simulink model "ppsim"  (R2024b)
settings: Solver=VariableStepAuto  StartTime=0.0  StopTime=10.0  RelTol=1e-3
values from neighbouring files (symbols this model uses):
  PpARMAXReg = ppc(tfarmax, ones(1, 4) * 0.3)    [main.m]
  PpARXReg = ppc(tfarx, ones(1, 4) * 0.3)    [main.m]
  PpDTFReg = ppc(dtf, ones(1, 4) * 0.1)    [main.m]
  usim = 1    [main.m]
  ut = [1 5]    [main.m]
undefined symbols (not defined in the file or in its folder): dtf, tfarmax, tfarx
settings Model: Creator=markminerov  LastModifiedBy=markminerov
settings DebuggingCC: AlgebraicLoopMsg=none

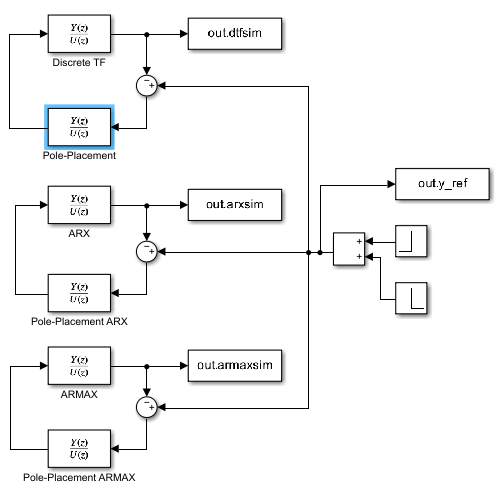
[thumbnail: Simulink's stored preview of the top-level diagram]
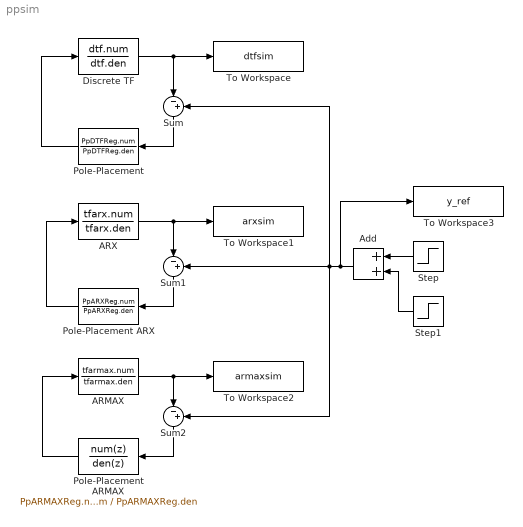
== system ppsim ==
  ARMAX : DiscreteTransferFcn  Numerator=tfarmax.num  Denominator=tfarmax.den
  ARX : DiscreteTransferFcn  Numerator=tfarx.num  Denominator=tfarx.den
  Add : Sum
  Discrete TF : DiscreteTransferFcn  Numerator=dtf.num  Denominator=dtf.den
  Pole-Placement : DiscreteTransferFcn  Numerator=PpDTFReg.num  Denominator=PpDTFReg.den
  Pole-Placement ARMAX : DiscreteTransferFcn  Numerator=PpARMAXReg.num  Denominator=PpARMAXReg.den
  Pole-Placement ARX : DiscreteTransferFcn  Numerator=PpARXReg.num  Denominator=PpARXReg.den
  Step : Step  Time=ut(1)  After=usim  SampleTime=0
  Step1 : Step  Time=ut(2)  After=-usim  SampleTime=0
  Sum : Sum  Inputs=|-+
  Sum1 : Sum  Inputs=|-+
  Sum2 : Sum  Inputs=|-+
  To Workspace : ToWorkspace  VariableName=dtfsim  SaveFormat=Timeseries  SampleTime=-1
  To Workspace1 : ToWorkspace  VariableName=arxsim  SaveFormat=Timeseries  SampleTime=-1
  To Workspace2 : ToWorkspace  VariableName=armaxsim  SaveFormat=Timeseries  SampleTime=-1
  To Workspace3 : ToWorkspace  VariableName=y_ref  SaveFormat=Timeseries  SampleTime=-1
  wires:
  Pole-Placement ARMAX/1 -> ARMAX/1
  Sum2/1 -> Pole-Placement ARMAX/1
  ARMAX/1 -> To Workspace2/1, Sum2/1
  Sum/1 -> Pole-Placement/1
  Sum1/1 -> Pole-Placement ARX/1
  Pole-Placement ARX/1 -> ARX/1
  Discrete TF/1 -> To Workspace/1, Sum/1
  Step/1 -> Add/1
  Step1/1 -> Add/2
  Add/1 -> To Workspace3/1, Sum2/2, Sum1/2, Sum/2
  Pole-Placement/1 -> Discrete TF/1
  ARX/1 -> Sum1/1, To Workspace1/1
